simulink model "huamo"  (R2014a)
settings: Solver=ode3  SolverMode=SingleTasking  StartTime=0.0  StopTime=10.0  RelTol=1e-3
PreLoadFcn:
  | waijung.modelPreload; % Required for working with Waijung Blockset. Do not remove.
undefined symbols (not defined in the file): ARM, dfilt, DiscIntNeverNeededParam, fdesignblkfcn, gcbh, Link, LQFP64, MDK, ST, STM32F405RG
libraries: simulink x33, stm32f4_io_lib x3, stm32f4_device_config_lib x2, dsparch4 x2
(part 5 of 6)

== system huamo/ from shangweiji/Enabled Subsystem6 ==
  P : Inport
  nP : Inport  Port=2
  nI : Inport  Port=3
  nD : Inport  Port=4
  status : Inport  Port=5
  Enable : EnablePort
  UART Tx : S-Function  Priority=1  FunctionName=stm32f4_usart  Parameters=configuration,uartmodule,transfer,baudrate,inputtype,outputtype,confstr,binheaderarray,binterminatorarray,asciiheader,asciiterminator,bindatalength,packetmode,varname,sampletime,sampletimestr,blockid  EnableBusSupport=off  mask(stm32f4_usart){configuration=Tx, uartmodule=1, baudrate=115200, databits=8, parity=No, stopbit=1, remaptxpin=Not used, remaprxpin=Not used, flowcontrol=None, remapctspin=Not used, remaprtspin=Not used, advanceoptions=off, rxbuffersize=512, txbuffersize=512, transfer=Non-Blocking, packetmode=Ascii, binheader='7E 7E', binterminator='03 03', porttype_double=0, porttype_single=0, porttype_int8=0, porttype_uint8=0, porttype_int16=0, porttype_uint16=0, porttype_int32=0, porttype_uint32=3, asciiformat='alt_change_OK', rx_asciiterminator=CRLF (0x0D 0x0A - "\r\n"), tx_asciiterminator=CRLF (0x0D 0x0A - "\r\n"), storagename=<empty>, varname=, inputtype=[0 ], outputtype=[0], binheaderarray=[0], binterminatorarray=[0], bindatalength=0, asciiheader='alt_change_OK\r\n', asciiterminator=[2 13 10], sampletime=-1, sampletimestr=0.005, blockid=fromshangweijiEnabledSubsystem6UARTTx, confstr=[ "dummy", "0", "*", "*", "0", "*", "*", "0", "*", "*", "0", "*", "*", "2", "4", "7", "2", "4", "2", "512", "512", "2", "1", "115200", "8", "No", "1", "None", "USART1"], lastmodule=1}
      mask prompts: uartmodule "UART Module"; baudrate "Baud rate (bps)"; databits "Data bits"; stopbit "Stop bit"; remaptxpin "Tx Pin"; remaprxpin "Rx Pin"; flowcontrol "Hardware flow control"; remapctspin "HW Flow control, CTS Pin"; remaprtspin "HW Flow control, RTS Pin"; advanceoptions "Advance options"; rxbuffersize "Rx buffer size (bytes)"; txbuffersize "Tx buffer size (bytes)"; packetmode "Packet mode"; binheader "Binary header (example: '7E 7E')"; binterminator "Binary terminator (example: '03 03')"; porttype_double "Number of data port, type DOUBLE"; porttype_single "Number of data port, type SINGLE"; porttype_int8 "Number of data port, type INT8"; porttype_uint8 "Number of data port, type UINT8"; porttype_int16 "Number of data port, type INT16"; porttype_uint16 "Number of data port, type UINT16"; porttype_int32 "Number of data port, type INT32"; porttype_uint32 "Number of data port, type UINT32"; asciiformat "Ascii format"; rx_asciiterminator "End of packet"; tx_asciiterminator "End of packet"; storagename "Buffer"; varname "Var name"; inputtype "Input data type"; outputtype "Output data type"; binheaderarray "Binary header"; binterminatorarray "Binary terminator"; bindatalength "Binary data length"; asciiheader "Ascii header (printf format)"; asciiterminator "Ascii terminator"; sampletime "Sample time (sec)"; sampletimestr "Compiled sample time (sec) in string"; confstr "Configuration string"; lastmodule "Last module selected"
      mask help:
      | Data type for Ascii format
      | %u, %i, %d, %o, %x: uint32
      | %e, %g, %f: single
      | %c: int8
      mask init:
      | stm32f4_usart_callback('init');
      mask Help: web(fullfile(waijungdocroot,'stm32f4_usart_tx.htm'), '-browser')
      mask TypeOptions configuration: Setup | Tx | Rx
      mask Callback configuration: stm32f4_usart_callback('configuration');
      mask TypeOptions uartmodule: 1 | 2 | 3 | 4 | 5 | 6
      mask Callback uartmodule: stm32f4_usart_callback('uartmodule');
      mask Callback baudrate: stm32f4_usart_callback('baudrate');
      mask TypeOptions databits: 8
      mask TypeOptions parity: No | Odd | Even
      mask TypeOptions stopbit: 0.5 | 1 | 1.5 | 2
      mask TypeOptions remaptxpin: Not used | A9 | B6
      mask TypeOptions remaprxpin: Not used | A10 | B7
      mask TypeOptions flowcontrol: None | RTS | CTS | RTS/CTS
      mask Callback flowcontrol: stm32f4_usart_callback('flowcontrol');
      mask TypeOptions remapctspin: Not used | A11
      mask TypeOptions remaprtspin: Not used | A12
      mask Callback advanceoptions: stm32f4_usart_callback('advanceoptions');
      mask TypeOptions rxbuffersize: 16 | 32 | 64 | 128 | 256 | 512 | 1024 | 2048
      mask TypeOptions txbuffersize: 16 | 32 | 64 | 128 | 256 | 512 | 1024 | 2048
      mask TypeOptions transfer: Blocking | Non-Blocking
      mask Callback transfer: stm32f4_usart_callback('transfer');
      mask TypeOptions packetmode: Ascii | Binary | Binary Vector | String Buffer
      mask Callback packetmode: stm32f4_usart_callback('packetmode');
      mask Callback binheader: stm32f4_usart_callback('binheader');
      mask Callback binterminator: stm32f4_usart_callback('binterminator');
      mask Callback porttype_double: stm32f4_usart_callback('porttype');
      mask Callback porttype_single: stm32f4_usart_callback('porttype');
      mask Callback porttype_int8: stm32f4_usart_callback('porttype');
      mask Callback porttype_uint8: stm32f4_usart_callback('porttype');
      mask Callback porttype_int16: stm32f4_usart_callback('porttype');
      mask Callback porttype_uint16: stm32f4_usart_callback('porttype');
      mask Callback porttype_int32: stm32f4_usart_callback('porttype');
      mask Callback porttype_uint32: stm32f4_usart_callback('porttype');
      mask Callback asciiformat: stm32f4_usart_callback('asciiformat');
      mask TypeOptions rx_asciiterminator: CR (0x0D - "\r") | LF (0x0A - "\n") | CRLF (0x0D 0x0A - "\r\n")
      mask Callback rx_asciiterminator: stm32f4_usart_callback('rx_asciiterminator');
      mask TypeOptions tx_asciiterminator: CR (0x0D - "\r") | LF (0x0A - "\n") | CRLF (0x0D 0x0A - "\r\n") | None
      mask Callback tx_asciiterminator: stm32f4_usart_callback('tx_asciiterminator');
      mask TypeOptions storagename: <empty>
      mask Callback storagename: stm32f4_usart_callback('storagename');
      mask Callback varname: stm32f4_usart_callback('varname');
      mask Callback sampletime: stm32f4_usart_callback('sampletime');
      mask Callback sampletimestr: stm32f4_usart_callback('sampletimestr');
      mask Callback blockid: stm32f4_usart_callback('blockid');
      mask Display: text(0.5, 0.5, 'Module: USART1_Tx\nPacket: Ascii\nTransfer: Non-Blocking\nTs (sec): 0.005','ver','middle','hor','center');
  Out1 : Outport
  Out2 : Outport  Port=2
  Out3 : Outport  Port=3
  Out4 : Outport  Port=4
  Out5 : Outport  Port=5
  wires:
  status/1 -> Out5/1
  nD/1 -> Out4/1
  nI/1 -> Out3/1
  nP/1 -> Out2/1
  P/1 -> Out1/1

== system huamo/Controller/Angle_hold ==
  Guidance_in : Inport
  Signal_back : Inport  Port=2
  parameter_roll : Inport  Port=3
  parameter_yaw : Inport  Port=4
  parameter_alt : Inport  Port=5
  alt_back : Inport  Port=6
  Enable : EnablePort
  Bus Selector : BusSelector  OutputSignals=thrust/CH3
  Constant1 : Constant  Value=[1;1;1;1]  OutDataTypeStr=single
  Gain : Gain  Gain=[1;1;1;1]  Multiplication=Matrix(K*u)
  If : If  IfExpression=u1 > 0.2
  Subsystem : Subsystem
  Sum : Sum  Inputs=|++
  Switch : Switch  Criteria=u2 > Threshold  Threshold=0.2
  Out1 : Outport
  Out2 : Outport  Port=2
  wires:
  Bus Selector/1 -> If/1, Gain/1, Switch/2  "<thrust/CH3>"
  Gain/1 -> Switch/3
  Constant1/1 -> Sum/2
  Sum/1 -> Out1/1
  Switch/1 -> Sum/1
  alt_back/1 -> Subsystem/1(In2)
  parameter_alt/1 -> Subsystem/2(In3)
  parameter_roll/1 -> Subsystem/3(In4)
  parameter_yaw/1 -> Subsystem/4(In5)
  Guidance_in/1 -> Bus Selector/1, Subsystem/5(In6)
  Signal_back/1 -> Subsystem/6(In7)
  Subsystem/1(Out1) -> Switch/1
  Subsystem/2(Out2) -> Out2/1
  If/1 -> Subsystem/Action

== system huamo/Controller/Parameter ==
  Mux : Mux  Inputs=5
  Mux1 : Mux  Inputs=5
  Mux2 : Mux  Inputs=5
  Out1 : Outport
  Out2 : Outport  Port=2
  Out3 : Outport  Port=3
  wires:
  [roll_nD] -> Mux/4
  [yaw_nD] -> Mux1/4
  [yaw_status] -> Mux1/5
  [roll_nI] -> Mux/3
  Mux/1 -> Out1/1
  [roll_nP] -> Mux/2
  [roll_status] -> Mux/5
  [yaw_nI] -> Mux1/3
  [roll_P] -> Mux/1
  [yaw_P] -> Mux1/1
  [yaw_nP] -> Mux1/2
  Mux1/1 -> Out2/1
  [alt_nD] -> Mux2/4
  [alt_status] -> Mux2/5
  [alt_nI] -> Mux2/3
  [alt_P] -> Mux2/1
  [alt_nP] -> Mux2/2
  Mux2/1 -> Out3/1

== system huamo/Controller/Velocity_Damper1 ==
  Signal_back : Inport
  status : Inport  Port=2
  Altitude_calculation : Subsystem
  Bus Selector1 : BusSelector  OutputSignals=angle,acceleration,altitude
  Constant : Constant  Value=[0 0 9.9]
  Controller : Subsystem
  Data Type Conversion1 : DataTypeConversion  OutDataTypeStr=single
  Data Type Conversion3 : DataTypeConversion  OutDataTypeStr=double
  Digital Clock : DigitalClock  SampleTime=-1
  Digital Clock1 : DigitalClock  SampleTime=-1
  Get_initial_altitude : MATLAB Function  TreatAsAtomicUnit=on
  Horizontal_velocity : Subsystem
  If : If  IfExpression=u1 > 2  ShowElse=off
  If Action Subsystem : Subsystem  TreatAsAtomicUnit=on
  MATLAB Function : MATLAB Function  TreatAsAtomicUnit=on
  accb_to_acce : Subsystem  TreatAsAtomicUnit=on
  Alt : Outport
  Alt_rate : Outport  Port=2
  M_y : Outport  Port=3
  M_x : Outport  Port=4
  wires:
  Signal_back/1 -> Bus Selector1/1
  Altitude_calculation/1(Out1) -> Data Type Conversion3/1, Controller/1(In1)
  Bus Selector1/1 -> accb_to_acce/1(angle)  "<angle>"
  Bus Selector1/2 -> accb_to_acce/2(accel)  "<acceleration>"
  Constant/1 -> accb_to_acce/3(bias_acc)
  Get_initial_altitude/1(y) -> Altitude_calculation/3(Basic_altitude)
  Digital Clock/1 -> Get_initial_altitude/2(t)
  If Action Subsystem/1(Out1) -> Altitude_calculation/Enable
  If/1 -> If Action Subsystem/Action
  Digital Clock1/1 -> If/1
  Bus Selector1/3 -> Get_initial_altitude/1(h), Altitude_calculation/2(Barometer)  "<altitude>"
  accb_to_acce/1(Out1) -> Horizontal_velocity/1(In1), Altitude_calculation/1(Accelerometer)
  Horizontal_velocity/1(Out1) -> M_y/1
  Horizontal_velocity/2(Out2) -> M_x/1
  Data Type Conversion3/1 -> MATLAB Function/2(u2)
  MATLAB Function/1(y) -> Data Type Conversion1/1
  status/1 -> MATLAB Function/1(u1)
  Controller/1(Out1) -> Alt_rate/1
  Data Type Conversion1/1 -> Alt/1

== system huamo/Controller/Velocity_Damper2 ==
  Signal_back : Inport
  status : Inport  Port=2
  Bus Selector1 : BusSelector  OutputSignals=alt
  Controller : Subsystem
  Data Type Conversion1 : DataTypeConversion  OutDataTypeStr=single
  Data Type Conversion3 : DataTypeConversion  OutDataTypeStr=double
  Lowpass Filter : Subsystem  DialogController=fdesignblkfcn  InitFcn=fdesignblkfcn(gcbh, {'InitFcn'});  mask(Lowpass Filter){}
      mask help: Design a lowpass filter
      settings: CopyFcn=fdesignblkfcn(gcbh, {'CopyFcn'});
      mask Help: helpview(mapfilelocation('dsp'), 'dsplowpassfilter');
      mask Display: disp('Lowpass')
  MATLAB Function : MATLAB Function  TreatAsAtomicUnit=on
  Rate Transition : RateTransition
  Alt : Outport
  Alt_rate : Outport  Port=2
  wires:
  Signal_back/1 -> Bus Selector1/1
  Bus Selector1/1 -> Rate Transition/1, Data Type Conversion3/1  "<alt>"
  Data Type Conversion3/1 -> MATLAB Function/2(u2)
  MATLAB Function/1(y) -> Lowpass Filter/1(In)
  status/1 -> MATLAB Function/1(u1)
  Controller/1(Out1) -> Alt_rate/1
  Data Type Conversion1/1 -> Alt/1
  Rate Transition/1 -> Controller/1(In1)
  Lowpass Filter/1(Out) -> Data Type Conversion1/1

== system huamo/Guidance_System/Duty to Force ==
  Duty : Inport
  Add : Sum  Inputs=+-
  Constant : Constant  OutDataTypeStr=single
  Gain : Gain  OutDataTypeStr=Inherit: Same as input
  Saturation : Saturate  UpperLimit=1  LowerLimit=0
  angle : Outport
  wires:
  Add/1 -> Gain/1
  Duty/1 -> Add/1
  Constant/1 -> Add/2
  Gain/1 -> Saturation/1
  Saturation/1 -> angle/1

== system huamo/Guidance_System/Duty to angle1 ==
  Duty : Inport
  Add : Sum  Inputs=+-
  Constant : Constant  Value=1.5  OutDataTypeStr=single
  Gain : Gain  Gain=-358  OutDataTypeStr=Inherit: Same as input
  Saturation : Saturate  UpperLimit=180  LowerLimit=-180
  angle : Outport
  wires:
  Add/1 -> Gain/1
  Duty/1 -> Add/1
  Constant/1 -> Add/2
  Gain/1 -> Saturation/1
  Saturation/1 -> angle/1

== system huamo/Guidance_System/Duty to angle2 ==
  Duty : Inport
  Add : Sum  Inputs=+-
  Constant : Constant  Value=1.5  OutDataTypeStr=single
  Gain : Gain  Gain=-40  OutDataTypeStr=Inherit: Same as input
  Saturation : Saturate  UpperLimit=25  LowerLimit=-25
  angle : Outport
  wires:
  Saturation/1 -> angle/1
  Gain/1 -> Saturation/1
  Constant/1 -> Add/2
  Duty/1 -> Add/1
  Add/1 -> Gain/1

== system huamo/Guidance_System/Duty to angle3 ==
  Duty : Inport
  Add : Sum  Inputs=+-
  Constant : Constant  Value=1.5  OutDataTypeStr=single
  Gain : Gain  Gain=40  OutDataTypeStr=Inherit: Same as input
  Saturation : Saturate  UpperLimit=25  LowerLimit=-25
  angle : Outport
  wires:
  Add/1 -> Gain/1
  Duty/1 -> Add/1
  Constant/1 -> Add/2
  Gain/1 -> Saturation/1
  Saturation/1 -> angle/1

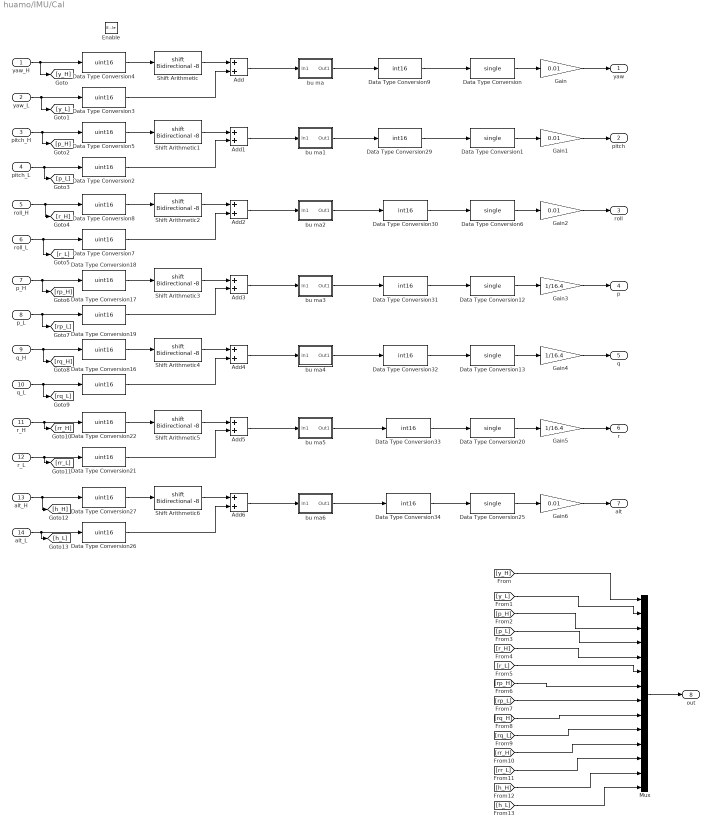
== system huamo/IMU/Cal ==
  yaw_H : Inport
  yaw_L : Inport  Port=2
  pitch_H : Inport  Port=3
  pitch_L : Inport  Port=4
  roll_H : Inport  Port=5
  roll_L : Inport  Port=6
  p_H : Inport  Port=7
  p_L : Inport  Port=8
  q_H : Inport  Port=9
  q_L : Inport  Port=10
  r_H : Inport  Port=11
  r_L : Inport  Port=12
  alt_H : Inport  Port=13
  alt_L : Inport  Port=14
  Enable : EnablePort
  Add{,1..6} (7 alike) : Sum  AccumDataTypeStr=uint16
  Data Type Conversion{,1,6,12..13,20,25} (7 alike) : DataTypeConversion  OutDataTypeStr=single
  Data Type Conversion{2..5,7..8,16..19,21..22,26..27} (14 alike) : DataTypeConversion  OutDataTypeStr=uint16
  Data Type Conversion{9,29..34} (7 alike) : DataTypeConversion  OutDataTypeStr=int16
  Gain{,1..2,6} (4 alike) : Gain  Gain=0.01
  Gain3 : Gain  Gain=1/16.4
  Gain4 : Gain  Gain=1/16.4
  Gain5 : Gain  Gain=1/16.4
  Mux : Mux  Inputs=14
  Shift Arithmetic{,1..6} (7 alike) : ArithShift  BitShiftNumber=-8
  bu ma : Subsystem
  bu ma1 : Subsystem
  bu ma2 : Subsystem
  bu ma3 : Subsystem
  bu ma4 : Subsystem
  bu ma5 : Subsystem
  bu ma6 : Subsystem
  yaw : Outport
  pitch : Outport  Port=2
  roll : Outport  Port=3
  p : Outport  Port=4
  q : Outport  Port=5
  r : Outport  Port=6
  alt : Outport  Port=7
  out : Outport  Port=8
  wires:
  Data Type Conversion/1 -> Gain/1
  yaw_H/1 -> [y_H], Data Type Conversion4/1
  yaw_L/1 -> [y_L], Data Type Conversion3/1
  Data Type Conversion1/1 -> Gain1/1
  pitch_H/1 -> [p_H], Data Type Conversion5/1
  pitch_L/1 -> [p_L], Data Type Conversion2/1
  Data Type Conversion4/1 -> Shift Arithmetic/1
  Data Type Conversion5/1 -> Shift Arithmetic1/1
  Data Type Conversion6/1 -> Gain2/1
  roll_H/1 -> [r_H], Data Type Conversion8/1
  roll_L/1 -> [r_L], Data Type Conversion7/1
  Data Type Conversion8/1 -> Shift Arithmetic2/1
  Gain/1 -> yaw/1
  Gain1/1 -> pitch/1
  Gain2/1 -> roll/1
  Data Type Conversion12/1 -> Gain3/1
  p_H/1 -> [rp_H], Data Type Conversion18/1
  p_L/1 -> [rp_L], Data Type Conversion17/1
  Data Type Conversion13/1 -> Gain4/1
  q_H/1 -> [rq_H], Data Type Conversion19/1
  q_L/1 -> [rq_L], Data Type Conversion16/1
  Data Type Conversion18/1 -> Shift Arithmetic3/1
  Data Type Conversion19/1 -> Shift Arithmetic4/1
  Data Type Conversion20/1 -> Gain5/1
  r_H/1 -> [rr_H], Data Type Conversion22/1
  r_L/1 -> [rr_L], Data Type Conversion21/1
  Data Type Conversion22/1 -> Shift Arithmetic5/1
  Gain3/1 -> p/1
  Gain4/1 -> q/1
  Gain5/1 -> r/1
  Data Type Conversion25/1 -> Gain6/1
  alt_H/1 -> [h_H], Data Type Conversion27/1
  alt_L/1 -> [h_L], Data Type Conversion26/1
  Data Type Conversion27/1 -> Shift Arithmetic6/1
  Gain6/1 -> alt/1
  Shift Arithmetic/1 -> Add/1
  Data Type Conversion3/1 -> Add/2
  Shift Arithmetic1/1 -> Add1/1
  Data Type Conversion2/1 -> Add1/2
  Shift Arithmetic2/1 -> Add2/1
  Data Type Conversion7/1 -> Add2/2
  Shift Arithmetic3/1 -> Add3/1
  Data Type Conversion17/1 -> Add3/2
  Shift Arithmetic4/1 -> Add4/1
  Data Type Conversion16/1 -> Add4/2
  Shift Arithmetic5/1 -> Add5/1
  Data Type Conversion21/1 -> Add5/2
  Shift Arithmetic6/1 -> Add6/1
  Data Type Conversion26/1 -> Add6/2
  Data Type Conversion29/1 -> Data Type Conversion1/1
  Data Type Conversion30/1 -> Data Type Conversion6/1
  Data Type Conversion31/1 -> Data Type Conversion12/1
  Data Type Conversion32/1 -> Data Type Conversion13/1
  Data Type Conversion33/1 -> Data Type Conversion20/1
  Data Type Conversion34/1 -> Data Type Conversion25/1
  Data Type Conversion9/1 -> Data Type Conversion/1
  Add/1 -> bu ma/1(In1)
  bu ma/1(Out1) -> Data Type Conversion9/1
  Add1/1 -> bu ma1/1(In1)
  bu ma1/1(Out1) -> Data Type Conversion29/1
  Add6/1 -> bu ma6/1(In1)
  bu ma6/1(Out1) -> Data Type Conversion34/1
  bu ma5/1(Out1) -> Data Type Conversion33/1
  bu ma4/1(Out1) -> Data Type Conversion32/1
  bu ma3/1(Out1) -> Data Type Conversion31/1
  bu ma2/1(Out1) -> Data Type Conversion30/1
  Add2/1 -> bu ma2/1(In1)
  Add3/1 -> bu ma3/1(In1)
  Add4/1 -> bu ma4/1(In1)
  Add5/1 -> bu ma5/1(In1)
  [y_H] -> Mux/1
  [y_L] -> Mux/2
  [p_H] -> Mux/3
  [p_L] -> Mux/4
  [r_H] -> Mux/5
  [r_L] -> Mux/6
  [rp_H] -> Mux/7
  [rp_L] -> Mux/8
  [rq_H] -> Mux/9
  [rq_L] -> Mux/10
  [rr_H] -> Mux/11
  [rr_L] -> Mux/12
  [h_H] -> Mux/13
  [h_L] -> Mux/14
  Mux/1 -> out/1

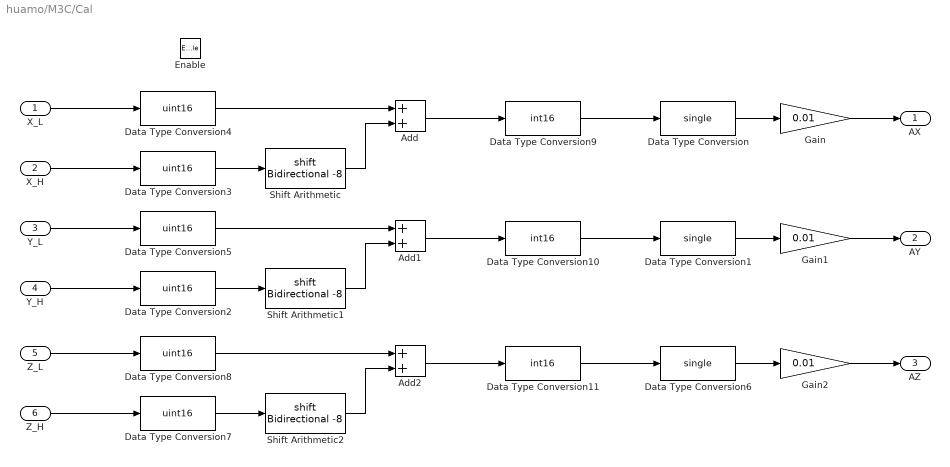
== system huamo/M3C/Cal ==
  X_L : Inport
  X_H : Inport  Port=2
  Y_L : Inport  Port=3
  Y_H : Inport  Port=4
  Z_L : Inport  Port=5
  Z_H : Inport  Port=6
  Enable : EnablePort
  Add : Sum  AccumDataTypeStr=uint16
  Add1 : Sum  AccumDataTypeStr=uint16
  Add2 : Sum  AccumDataTypeStr=uint16
  Data Type Conversion : DataTypeConversion  OutDataTypeStr=single
  Data Type Conversion1 : DataTypeConversion  OutDataTypeStr=single
  Data Type Conversion10 : DataTypeConversion  OutDataTypeStr=int16
  Data Type Conversion11 : DataTypeConversion  OutDataTypeStr=int16
  Data Type Conversion{2..5,7..8} (6 alike) : DataTypeConversion  OutDataTypeStr=uint16
  Data Type Conversion6 : DataTypeConversion  OutDataTypeStr=single
  Data Type Conversion9 : DataTypeConversion  OutDataTypeStr=int16
  Gain : Gain  Gain=0.01
  Gain1 : Gain  Gain=0.01
  Gain2 : Gain  Gain=0.01
  Shift Arithmetic : ArithShift  BitShiftNumber=-8
  Shift Arithmetic1 : ArithShift  BitShiftNumber=-8
  Shift Arithmetic2 : ArithShift  BitShiftNumber=-8
  AX : Outport
  AY : Outport  Port=2
  AZ : Outport  Port=3
  wires:
  Data Type Conversion/1 -> Gain/1
  Shift Arithmetic/1 -> Add/2
  X_L/1 -> Data Type Conversion4/1
  X_H/1 -> Data Type Conversion3/1
  Data Type Conversion3/1 -> Shift Arithmetic/1
  Add/1 -> Data Type Conversion9/1
  Data Type Conversion1/1 -> Gain1/1
  Shift Arithmetic1/1 -> Add1/2
  Y_L/1 -> Data Type Conversion5/1
  Y_H/1 -> Data Type Conversion2/1
  Data Type Conversion2/1 -> Shift Arithmetic1/1
  Add1/1 -> Data Type Conversion10/1
  Data Type Conversion4/1 -> Add/1
  Data Type Conversion5/1 -> Add1/1
  Data Type Conversion6/1 -> Gain2/1
  Shift Arithmetic2/1 -> Add2/2
  Z_L/1 -> Data Type Conversion8/1
  Z_H/1 -> Data Type Conversion7/1
  Data Type Conversion7/1 -> Shift Arithmetic2/1
  Add2/1 -> Data Type Conversion11/1
  Data Type Conversion8/1 -> Add2/1
  Gain/1 -> AX/1
  Gain1/1 -> AY/1
  Gain2/1 -> AZ/1
  Data Type Conversion9/1 -> Data Type Conversion/1
  Data Type Conversion10/1 -> Data Type Conversion1/1
  Data Type Conversion11/1 -> Data Type Conversion6/1

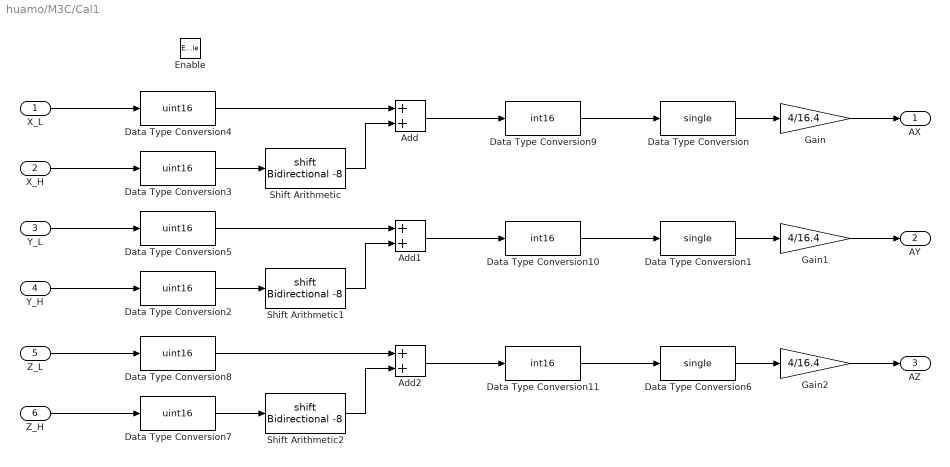
== system huamo/M3C/Cal1 ==
  X_L : Inport
  X_H : Inport  Port=2
  Y_L : Inport  Port=3
  Y_H : Inport  Port=4
  Z_L : Inport  Port=5
  Z_H : Inport  Port=6
  Enable : EnablePort
  Add : Sum  AccumDataTypeStr=uint16
  Add1 : Sum  AccumDataTypeStr=uint16
  Add2 : Sum  AccumDataTypeStr=uint16
  Data Type Conversion : DataTypeConversion  OutDataTypeStr=single
  Data Type Conversion1 : DataTypeConversion  OutDataTypeStr=single
  Data Type Conversion10 : DataTypeConversion  OutDataTypeStr=int16
  Data Type Conversion11 : DataTypeConversion  OutDataTypeStr=int16
  Data Type Conversion{2..5,7..8} (6 alike) : DataTypeConversion  OutDataTypeStr=uint16
  Data Type Conversion6 : DataTypeConversion  OutDataTypeStr=single
  Data Type Conversion9 : DataTypeConversion  OutDataTypeStr=int16
  Gain : Gain  Gain=4/16.4
  Gain1 : Gain  Gain=4/16.4
  Gain2 : Gain  Gain=4/16.4
  Shift Arithmetic : ArithShift  BitShiftNumber=-8
  Shift Arithmetic1 : ArithShift  BitShiftNumber=-8
  Shift Arithmetic2 : ArithShift  BitShiftNumber=-8
  AX : Outport
  AY : Outport  Port=2
  AZ : Outport  Port=3
  wires:
  Data Type Conversion11/1 -> Data Type Conversion6/1
  Data Type Conversion10/1 -> Data Type Conversion1/1
  Data Type Conversion9/1 -> Data Type Conversion/1
  Gain2/1 -> AZ/1
  Gain1/1 -> AY/1
  Gain/1 -> AX/1
  Data Type Conversion8/1 -> Add2/1
  Add2/1 -> Data Type Conversion11/1
  Data Type Conversion7/1 -> Shift Arithmetic2/1
  Z_H/1 -> Data Type Conversion7/1
  Z_L/1 -> Data Type Conversion8/1
  Shift Arithmetic2/1 -> Add2/2
  Data Type Conversion6/1 -> Gain2/1
  Data Type Conversion5/1 -> Add1/1
  Data Type Conversion4/1 -> Add/1
  Add1/1 -> Data Type Conversion10/1
  Data Type Conversion2/1 -> Shift Arithmetic1/1
  Y_H/1 -> Data Type Conversion2/1
  Y_L/1 -> Data Type Conversion5/1
  Shift Arithmetic1/1 -> Add1/2
  Data Type Conversion1/1 -> Gain1/1
  Add/1 -> Data Type Conversion9/1
  Data Type Conversion3/1 -> Shift Arithmetic/1
  X_H/1 -> Data Type Conversion3/1
  X_L/1 -> Data Type Conversion4/1
  Shift Arithmetic/1 -> Add/2
  Data Type Conversion/1 -> Gain/1

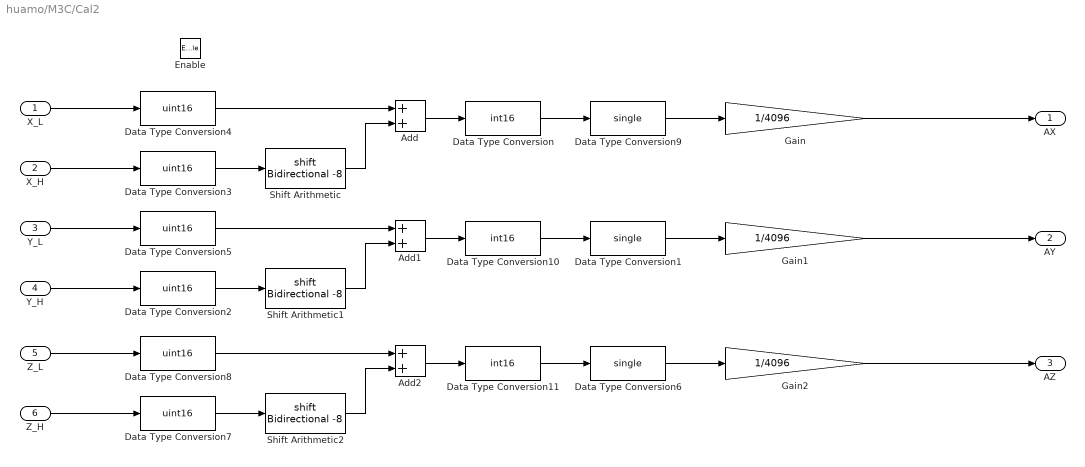
== system huamo/M3C/Cal2 ==
  X_L : Inport
  X_H : Inport  Port=2
  Y_L : Inport  Port=3
  Y_H : Inport  Port=4
  Z_L : Inport  Port=5
  Z_H : Inport  Port=6
  Enable : EnablePort
  Add : Sum
  Add1 : Sum
  Add2 : Sum
  Data Type Conversion : DataTypeConversion  OutDataTypeStr=int16
  Data Type Conversion1 : DataTypeConversion  OutDataTypeStr=single
  Data Type Conversion10 : DataTypeConversion  OutDataTypeStr=int16
  Data Type Conversion11 : DataTypeConversion  OutDataTypeStr=int16
  Data Type Conversion{2..5,7..8} (6 alike) : DataTypeConversion  OutDataTypeStr=uint16
  Data Type Conversion6 : DataTypeConversion  OutDataTypeStr=single
  Data Type Conversion9 : DataTypeConversion  OutDataTypeStr=single
  Gain : Gain  Gain=1/4096
  Gain1 : Gain  Gain=1/4096
  Gain2 : Gain  Gain=1/4096
  Shift Arithmetic : ArithShift  BitShiftNumber=-8
  Shift Arithmetic1 : ArithShift  BitShiftNumber=-8
  Shift Arithmetic2 : ArithShift  BitShiftNumber=-8
  AX : Outport
  AY : Outport  Port=2
  AZ : Outport  Port=3
  wires:
  Shift Arithmetic/1 -> Add/2
  X_L/1 -> Data Type Conversion4/1
  X_H/1 -> Data Type Conversion3/1
  Data Type Conversion3/1 -> Shift Arithmetic/1
  Add/1 -> Data Type Conversion/1
  Shift Arithmetic1/1 -> Add1/2
  Y_L/1 -> Data Type Conversion5/1
  Y_H/1 -> Data Type Conversion2/1
  Data Type Conversion2/1 -> Shift Arithmetic1/1
  Add1/1 -> Data Type Conversion10/1
  Data Type Conversion4/1 -> Add/1
  Data Type Conversion5/1 -> Add1/1
  Shift Arithmetic2/1 -> Add2/2
  Z_L/1 -> Data Type Conversion8/1
  Z_H/1 -> Data Type Conversion7/1
  Data Type Conversion7/1 -> Shift Arithmetic2/1
  Add2/1 -> Data Type Conversion11/1
  Data Type Conversion8/1 -> Add2/1
  Data Type Conversion/1 -> Data Type Conversion9/1
  Data Type Conversion1/1 -> Gain1/1
  Data Type Conversion6/1 -> Gain2/1
  Data Type Conversion9/1 -> Gain/1
  Data Type Conversion10/1 -> Data Type Conversion1/1
  Data Type Conversion11/1 -> Data Type Conversion6/1
  Gain/1 -> AX/1
  Gain1/1 -> AY/1
  Gain2/1 -> AZ/1

== system huamo/M3C/Cal3 ==
  L : Inport
  LH : Inport  Port=2
  HL : Inport  Port=3
  H : Inport  Port=4
  Enable : EnablePort
  Add : Sum  Inputs=++++
  Data Type Conversion : DataTypeConversion  OutDataTypeStr=int32
  Data Type Conversion{2..5} (4 alike) : DataTypeConversion  OutDataTypeStr=uint16
  Data Type Conversion9 : DataTypeConversion  OutDataTypeStr=single
  Gain : Gain  Gain=0.01
  Shift Arithmetic : ArithShift  BitShiftNumber=-8
  Shift Arithmetic1 : ArithShift  BitShiftNumber=-8
  Shift Arithmetic2 : ArithShift  BitShiftNumber=-8
  Altitude : Outport
  wires:
  Gain/1 -> Altitude/1
  Data Type Conversion9/1 -> Gain/1
  Data Type Conversion/1 -> Data Type Conversion9/1
  Data Type Conversion4/1 -> Add/1
  Data Type Conversion2/1 -> Shift Arithmetic1/1
  H/1 -> Data Type Conversion2/1
  HL/1 -> Data Type Conversion5/1
  Add/1 -> Data Type Conversion/1
  Data Type Conversion3/1 -> Shift Arithmetic/1
  LH/1 -> Data Type Conversion3/1
  L/1 -> Data Type Conversion4/1
  Shift Arithmetic/1 -> Add/2
  Data Type Conversion5/1 -> Shift Arithmetic2/1
  Shift Arithmetic2/1 -> Add/3
  Shift Arithmetic1/1 -> Add/4

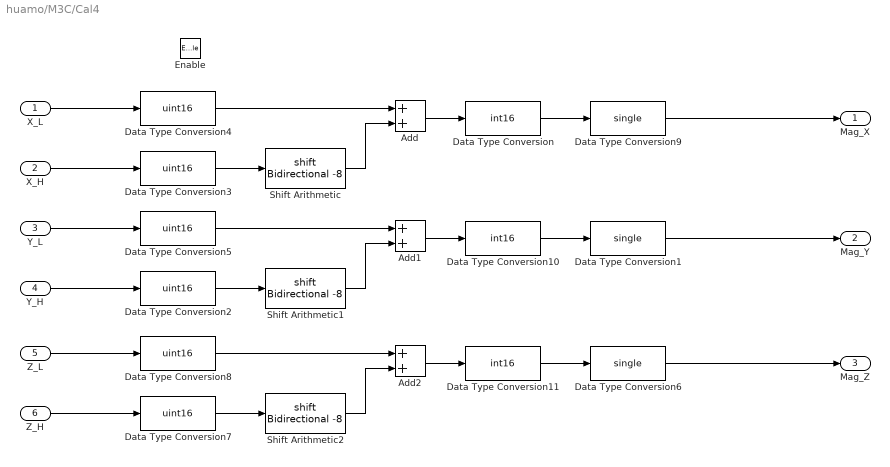
== system huamo/M3C/Cal4 ==
  X_L : Inport
  X_H : Inport  Port=2
  Y_L : Inport  Port=3
  Y_H : Inport  Port=4
  Z_L : Inport  Port=5
  Z_H : Inport  Port=6
  Enable : EnablePort
  Add : Sum
  Add1 : Sum
  Add2 : Sum
  Data Type Conversion : DataTypeConversion  OutDataTypeStr=int16
  Data Type Conversion1 : DataTypeConversion  OutDataTypeStr=single
  Data Type Conversion10 : DataTypeConversion  OutDataTypeStr=int16
  Data Type Conversion11 : DataTypeConversion  OutDataTypeStr=int16
  Data Type Conversion{2..5,7..8} (6 alike) : DataTypeConversion  OutDataTypeStr=uint16
  Data Type Conversion6 : DataTypeConversion  OutDataTypeStr=single
  Data Type Conversion9 : DataTypeConversion  OutDataTypeStr=single
  Shift Arithmetic : ArithShift  BitShiftNumber=-8
  Shift Arithmetic1 : ArithShift  BitShiftNumber=-8
  Shift Arithmetic2 : ArithShift  BitShiftNumber=-8
  Mag_X : Outport
  Mag_Y : Outport  Port=2
  Mag_Z : Outport  Port=3
  wires:
  Shift Arithmetic/1 -> Add/2
  X_L/1 -> Data Type Conversion4/1
  X_H/1 -> Data Type Conversion3/1
  Data Type Conversion3/1 -> Shift Arithmetic/1
  Add/1 -> Data Type Conversion/1
  Shift Arithmetic1/1 -> Add1/2
  Y_L/1 -> Data Type Conversion5/1
  Y_H/1 -> Data Type Conversion2/1
  Data Type Conversion2/1 -> Shift Arithmetic1/1
  Add1/1 -> Data Type Conversion10/1
  Data Type Conversion4/1 -> Add/1
  Data Type Conversion5/1 -> Add1/1
  Shift Arithmetic2/1 -> Add2/2
  Z_L/1 -> Data Type Conversion8/1
  Z_H/1 -> Data Type Conversion7/1
  Data Type Conversion7/1 -> Shift Arithmetic2/1
  Add2/1 -> Data Type Conversion11/1
  Data Type Conversion8/1 -> Add2/1
  Data Type Conversion/1 -> Data Type Conversion9/1
  Data Type Conversion1/1 -> Mag_Y/1
  Data Type Conversion6/1 -> Mag_Z/1
  Data Type Conversion10/1 -> Data Type Conversion1/1
  Data Type Conversion11/1 -> Data Type Conversion6/1
  Data Type Conversion9/1 -> Mag_X/1

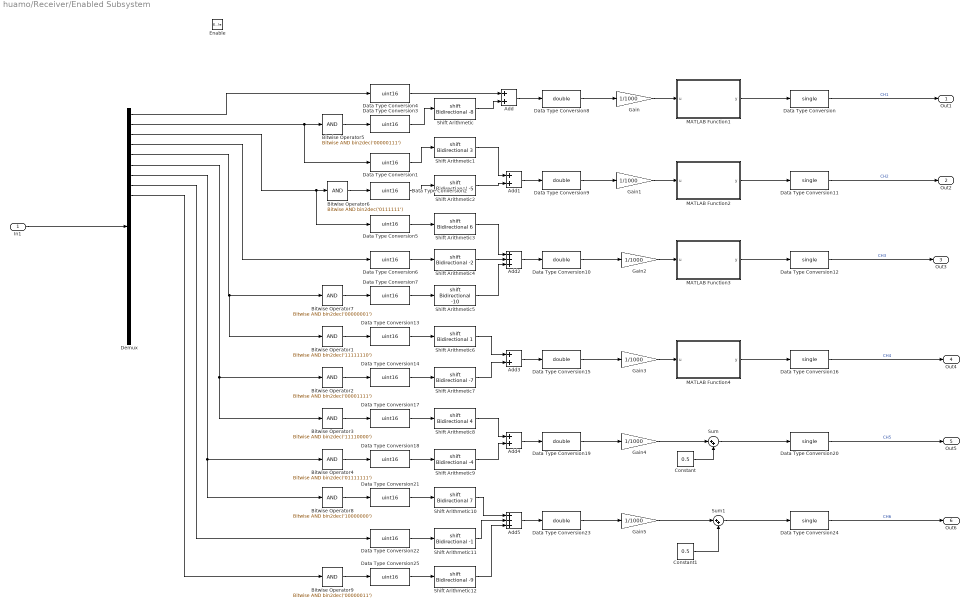
== system huamo/Receiver/Enabled Subsystem ==
  In1 : Inport
  Enable : EnablePort
  Add{,1,3..4} (4 alike) : Sum  AccumDataTypeStr=uint16
  Add2 : Sum  Inputs=+++  AccumDataTypeStr=uint16
  Add5 : Sum  Inputs=+++  AccumDataTypeStr=uint16
  Bitwise Operator1 : simulink/Logic and Bit Operations/Bitwise Operator  logicop=AND  UseBitMask=on  BitMask=bin2dec('11111110')  BitMaskRealWorld=Stored Integer
  Bitwise Operator2 : simulink/Logic and Bit Operations/Bitwise Operator  logicop=AND  UseBitMask=on  BitMask=bin2dec('00001111')  BitMaskRealWorld=Stored Integer
  Bitwise Operator3 : simulink/Logic and Bit Operations/Bitwise Operator  logicop=AND  UseBitMask=on  BitMask=bin2dec('11110000')  BitMaskRealWorld=Stored Integer
  Bitwise Operator4 : simulink/Logic and Bit Operations/Bitwise Operator  logicop=AND  UseBitMask=on  BitMask=bin2dec('01111111')  BitMaskRealWorld=Stored Integer
  Bitwise Operator5 : simulink/Logic and Bit Operations/Bitwise Operator  logicop=AND  UseBitMask=on  BitMask=bin2dec('00000111')  BitMaskRealWorld=Stored Integer
  Bitwise Operator6 : simulink/Logic and Bit Operations/Bitwise Operator  logicop=AND  UseBitMask=on  BitMask=bin2dec('0111111')  BitMaskRealWorld=Stored Integer
  Bitwise Operator7 : simulink/Logic and Bit Operations/Bitwise Operator  logicop=AND  UseBitMask=on  BitMask=bin2dec('00000001')  BitMaskRealWorld=Stored Integer
  Bitwise Operator8 : simulink/Logic and Bit Operations/Bitwise Operator  logicop=AND  UseBitMask=on  BitMask=bin2dec('10000000')  BitMaskRealWorld=Stored Integer
  Bitwise Operator9 : simulink/Logic and Bit Operations/Bitwise Operator  logicop=AND  UseBitMask=on  BitMask=bin2dec('00000011')  BitMaskRealWorld=Stored Integer
  Constant : Constant  Value=0.5
  Constant1 : Constant  Value=0.5
  Data Type Conversion{,11..12,16,20,24} (6 alike) : DataTypeConversion  OutDataTypeStr=single
  Data Type Conversion{1..7,13..14,17..18,21..22,25} (14 alike) : DataTypeConversion  OutDataTypeStr=uint16
  Data Type Conversion{8..10,15,19,23} (6 alike) : DataTypeConversion  OutDataTypeStr=double
  Demux : Demux  Outputs=23
  Gain{,1..5} (6 alike) : Gain  Gain=1/1000
  MATLAB Function1 : MATLAB Function  TreatAsAtomicUnit=on
  MATLAB Function2 : MATLAB Function  TreatAsAtomicUnit=on
  MATLAB Function3 : MATLAB Function  TreatAsAtomicUnit=on
  MATLAB Function4 : MATLAB Function  TreatAsAtomicUnit=on
  Shift Arithmetic : ArithShift  BitShiftNumber=-8
  Shift Arithmetic1 : ArithShift  BitShiftNumber=3
  Shift Arithmetic10 : ArithShift  BitShiftNumber=7
  Shift Arithmetic11 : ArithShift  BitShiftNumber=-1
  Shift Arithmetic12 : ArithShift  BitShiftNumber=-9
  Shift Arithmetic2 : ArithShift  BitShiftNumber=-5
  Shift Arithmetic3 : ArithShift  BitShiftNumber=6
  Shift Arithmetic4 : ArithShift  BitShiftNumber=-2
  Shift Arithmetic5 : ArithShift  BitShiftNumber=-10
  Shift Arithmetic6 : ArithShift  BitShiftNumber=1
  Shift Arithmetic7 : ArithShift  BitShiftNumber=-7
  Shift Arithmetic8 : ArithShift  BitShiftNumber=4
  Shift Arithmetic9 : ArithShift  BitShiftNumber=-4
  Sum : Sum  Inputs=|++
  Sum1 : Sum  Inputs=|++
  Out1 : Outport
  Out2 : Outport  Port=2
  Out3 : Outport  Port=3
  Out4 : Outport  Port=4
  Out5 : Outport  Port=5
  Out6 : Outport  Port=6
  wires:
  Data Type Conversion4/1 -> Add/1
  Data Type Conversion3/1 -> Shift Arithmetic/1
  Shift Arithmetic/1 -> Add/2
  Demux/1 -> Data Type Conversion4/1
  Bitwise Operator5/1 -> Data Type Conversion3/1
  Data Type Conversion1/1 -> Shift Arithmetic1/1
  Demux/2 -> Data Type Conversion1/1, Bitwise Operator5/1
  Data Type Conversion2/1 -> Shift Arithmetic2/1
  Shift Arithmetic1/1 -> Add1/1
  Shift Arithmetic2/1 -> Add1/2
  Data Type Conversion5/1 -> Shift Arithmetic3/1
  Demux/4 -> Data Type Conversion6/1
  Data Type Conversion6/1 -> Shift Arithmetic4/1
  Data Type Conversion7/1 -> Shift Arithmetic5/1
  Shift Arithmetic3/1 -> Add2/1
  Shift Arithmetic4/1 -> Add2/2
  Shift Arithmetic5/1 -> Add2/3
  Add1/1 -> Data Type Conversion9/1
  Add2/1 -> Data Type Conversion10/1
  Data Type Conversion10/1 -> Gain2/1
  Gain/1 -> MATLAB Function1/1(u)
  Gain1/1 -> MATLAB Function2/1(u)
  Gain2/1 -> MATLAB Function3/1(u)
  Data Type Conversion/1 -> Out1/1  "CH1"
  Data Type Conversion11/1 -> Out2/1  "CH2"
  Data Type Conversion12/1 -> Out3/1  "CH3"
  In1/1 -> Demux/1
  Demux/3 -> Bitwise Operator6/1, Data Type Conversion5/1
  Bitwise Operator6/1 -> Data Type Conversion2/1
  Bitwise Operator7/1 -> Data Type Conversion7/1
  Demux/5 -> Bitwise Operator1/1, Bitwise Operator7/1
  Bitwise Operator1/1 -> Data Type Conversion13/1
  Data Type Conversion13/1 -> Shift Arithmetic6/1
  Demux/6 -> Bitwise Operator3/1, Bitwise Operator2/1
  Bitwise Operator2/1 -> Data Type Conversion14/1
  Data Type Conversion14/1 -> Shift Arithmetic7/1
  Shift Arithmetic6/1 -> Add3/1
  Shift Arithmetic7/1 -> Add3/2
  Add3/1 -> Data Type Conversion15/1
  Data Type Conversion15/1 -> Gain3/1
  Gain3/1 -> MATLAB Function4/1(u)
  Bitwise Operator3/1 -> Data Type Conversion17/1
  Data Type Conversion17/1 -> Shift Arithmetic8/1
  Bitwise Operator4/1 -> Data Type Conversion18/1
  Data Type Conversion18/1 -> Shift Arithmetic9/1
  Shift Arithmetic8/1 -> Add4/1
  Shift Arithmetic9/1 -> Add4/2
  Add4/1 -> Data Type Conversion19/1
  Demux/7 -> Bitwise Operator8/1, Bitwise Operator4/1
  Data Type Conversion19/1 -> Gain4/1
  Bitwise Operator8/1 -> Data Type Conversion21/1
  Data Type Conversion21/1 -> Shift Arithmetic10/1
  Demux/8 -> Data Type Conversion22/1
  Data Type Conversion22/1 -> Shift Arithmetic11/1
  Shift Arithmetic10/1 -> Add5/1
  Shift Arithmetic11/1 -> Add5/2
  Add5/1 -> Data Type Conversion23/1
  Data Type Conversion23/1 -> Gain5/1
  Data Type Conversion25/1 -> Shift Arithmetic12/1
  Shift Arithmetic12/1 -> Add5/3
  Bitwise Operator9/1 -> Data Type Conversion25/1
  Demux/9 -> Bitwise Operator9/1
  Data Type Conversion16/1 -> Out4/1  "CH4"
  Data Type Conversion20/1 -> Out5/1  "CH5"
  Data Type Conversion24/1 -> Out6/1  "CH6"
  Add/1 -> Data Type Conversion8/1
  Data Type Conversion8/1 -> Gain/1
  Data Type Conversion9/1 -> Gain1/1
  MATLAB Function1/1(y) -> Data Type Conversion/1
  MATLAB Function4/1(y) -> Data Type Conversion16/1
  MATLAB Function2/1(y) -> Data Type Conversion11/1
  Gain4/1 -> Sum/1
  Sum/1 -> Data Type Conversion20/1
  Constant/1 -> Sum/2
  Sum1/1 -> Data Type Conversion24/1
  Gain5/1 -> Sum1/1
  Constant1/1 -> Sum1/2
  MATLAB Function3/1(y) -> Data Type Conversion12/1

== system huamo/to shangweiji/Subsystem ==
  In3 : Inport
  Demux : Demux  Outputs=5
  UART Tx : S-Function  Priority=1  FunctionName=stm32f4_usart  Parameters=configuration,uartmodule,transfer,baudrate,inputtype,outputtype,confstr,binheaderarray,binterminatorarray,asciiheader,asciiterminator,bindatalength,packetmode,varname,sampletime,sampletimestr,blockid  EnableBusSupport=off  mask(stm32f4_usart){configuration=Tx, uartmodule=1, baudrate=115200, databits=8, parity=No, stopbit=1, remaptxpin=Not used, remaprxpin=Not used, flowcontrol=None, remapctspin=Not used, remaprtspin=Not used, advanceoptions=off, rxbuffersize=512, txbuffersize=512, transfer=Non-Blocking, packetmode=Ascii, binheader='7E 7E', binterminator='03 03', porttype_double=0, porttype_single=0, porttype_int8=0, porttype_uint8=23, porttype_int16=0, porttype_uint16=0, porttype_int32=0, porttype_uint32=0, asciiformat='dianji=%f,%f,%f,%f,%f', rx_asciiterminator=CRLF (0x0D 0x0A - "\r\n"), tx_asciiterminator=CRLF (0x0D 0x0A - "\r\n"), storagename=<empty>, varname=, inputtype=[5  1 1 1 1 1], outputtype=[0], binheaderarray=[0], binterminatorarray=[0], bindatalength=0, asciiheader='dianji=%f,%f,%f,%f,%f\r\n', asciiterminator=[2 13 10], sampletime=-1, sampletimestr=0.6, blockid=toshangweijiSubsystemUARTTx, confstr=[ "dummy", "0", "*", "*", "0", "*", "*", "0", "*", "*", "0", "*", "*", "2", "4", "7", "2", "4", "2", "512", "512", "2", "1", "115200", "8", "No", "1", "None", "USART1"], lastmodule=1}
      mask prompts: uartmodule "UART Module"; baudrate "Baud rate (bps)"; databits "Data bits"; stopbit "Stop bit"; remaptxpin "Tx Pin"; remaprxpin "Rx Pin"; flowcontrol "Hardware flow control"; remapctspin "HW Flow control, CTS Pin"; remaprtspin "HW Flow control, RTS Pin"; advanceoptions "Advance options"; rxbuffersize "Rx buffer size (bytes)"; txbuffersize "Tx buffer size (bytes)"; packetmode "Packet mode"; binheader "Binary header (example: '7E 7E')"; binterminator "Binary terminator (example: '03 03')"; porttype_double "Number of data port, type DOUBLE"; porttype_single "Number of data port, type SINGLE"; porttype_int8 "Number of data port, type INT8"; porttype_uint8 "Number of data port, type UINT8"; porttype_int16 "Number of data port, type INT16"; porttype_uint16 "Number of data port, type UINT16"; porttype_int32 "Number of data port, type INT32"; porttype_uint32 "Number of data port, type UINT32"; asciiformat "Ascii format"; rx_asciiterminator "End of packet"; tx_asciiterminator "End of packet"; storagename "Buffer"; varname "Var name"; inputtype "Input data type"; outputtype "Output data type"; binheaderarray "Binary header"; binterminatorarray "Binary terminator"; bindatalength "Binary data length"; asciiheader "Ascii header (printf format)"; asciiterminator "Ascii terminator"; sampletime "Sample time (sec)"; sampletimestr "Compiled sample time (sec) in string"; confstr "Configuration string"; lastmodule "Last module selected"
      mask help:
      | Data type for Ascii format
      | %u, %i, %d, %o, %x: uint32
      | %e, %g, %f: single
      | %c: int8
      mask init:
      | stm32f4_usart_callback('init');
      mask Help: web(fullfile(waijungdocroot,'stm32f4_usart_tx.htm'), '-browser')
      mask TypeOptions configuration: Setup | Tx | Rx
      mask Callback configuration: stm32f4_usart_callback('configuration');
      mask TypeOptions uartmodule: 1 | 2 | 3 | 4 | 5 | 6
      mask Callback uartmodule: stm32f4_usart_callback('uartmodule');
      mask Callback baudrate: stm32f4_usart_callback('baudrate');
      mask TypeOptions databits: 8
      mask TypeOptions parity: No | Odd | Even
      mask TypeOptions stopbit: 0.5 | 1 | 1.5 | 2
      mask TypeOptions remaptxpin: Not used | A9 | B6
      mask TypeOptions remaprxpin: Not used | A10 | B7
      mask TypeOptions flowcontrol: None | RTS | CTS | RTS/CTS
      mask Callback flowcontrol: stm32f4_usart_callback('flowcontrol');
      mask TypeOptions remapctspin: Not used | A11
      mask TypeOptions remaprtspin: Not used | A12
      mask Callback advanceoptions: stm32f4_usart_callback('advanceoptions');
      mask TypeOptions rxbuffersize: 16 | 32 | 64 | 128 | 256 | 512 | 1024 | 2048
      mask TypeOptions txbuffersize: 16 | 32 | 64 | 128 | 256 | 512 | 1024 | 2048
      mask TypeOptions transfer: Blocking | Non-Blocking
      mask Callback transfer: stm32f4_usart_callback('transfer');
      mask TypeOptions packetmode: Ascii | Binary | Binary Vector | String Buffer
      mask Callback packetmode: stm32f4_usart_callback('packetmode');
      mask Callback binheader: stm32f4_usart_callback('binheader');
      mask Callback binterminator: stm32f4_usart_callback('binterminator');
      mask Callback porttype_double: stm32f4_usart_callback('porttype');
      mask Callback porttype_single: stm32f4_usart_callback('porttype');
      mask Callback porttype_int8: stm32f4_usart_callback('porttype');
      mask Callback porttype_uint8: stm32f4_usart_callback('porttype');
      mask Callback porttype_int16: stm32f4_usart_callback('porttype');
      mask Callback porttype_uint16: stm32f4_usart_callback('porttype');
      mask Callback porttype_int32: stm32f4_usart_callback('porttype');
      mask Callback porttype_uint32: stm32f4_usart_callback('porttype');
      mask Callback asciiformat: stm32f4_usart_callback('asciiformat');
      mask TypeOptions rx_asciiterminator: CR (0x0D - "\r") | LF (0x0A - "\n") | CRLF (0x0D 0x0A - "\r\n")
      mask Callback rx_asciiterminator: stm32f4_usart_callback('rx_asciiterminator');
      mask TypeOptions tx_asciiterminator: CR (0x0D - "\r") | LF (0x0A - "\n") | CRLF (0x0D 0x0A - "\r\n") | None
      mask Callback tx_asciiterminator: stm32f4_usart_callback('tx_asciiterminator');
      mask TypeOptions storagename: <empty>
      mask Callback storagename: stm32f4_usart_callback('storagename');
      mask Callback varname: stm32f4_usart_callback('varname');
      mask Callback sampletime: stm32f4_usart_callback('sampletime');
      mask Callback sampletimestr: stm32f4_usart_callback('sampletimestr');
      mask Callback blockid: stm32f4_usart_callback('blockid');
      mask Display: text(0.5, 0.5, 'Module: USART1_Tx\nPacket: Ascii\nTransfer: Non-Blocking\nTs (sec): 0.6','ver','middle','hor','center'); port_label('input', 1,'single'); port_label('input', 2,'single'); port_label('input', 3,'single'); port_label('input', 4,'single'); port_label('input', 5,'single');
  wires:
  Demux/1 -> UART Tx/1
  Demux/2 -> UART Tx/2
  Demux/3 -> UART Tx/3
  Demux/4 -> UART Tx/4
  In3/1 -> Demux/1
  Demux/5 -> UART Tx/5

== system huamo/ from shangweiji/Enabled Subsystem1/If Action Subsystem ==
  Action Port : ActionPort  ActionType=then
  UART Tx : S-Function  Priority=1  FunctionName=stm32f4_usart  Parameters=configuration,uartmodule,transfer,baudrate,inputtype,outputtype,confstr,binheaderarray,binterminatorarray,asciiheader,asciiterminator,bindatalength,packetmode,varname,sampletime,sampletimestr,blockid  EnableBusSupport=off  mask(stm32f4_usart){configuration=Tx, uartmodule=1, baudrate=115200, databits=8, parity=No, stopbit=1, remaptxpin=Not used, remaprxpin=Not used, flowcontrol=None, remapctspin=Not used, remaprtspin=Not used, advanceoptions=off, rxbuffersize=512, txbuffersize=512, transfer=Non-Blocking, packetmode=Ascii, binheader='7E 7E', binterminator='03 03', porttype_double=0, porttype_single=0, porttype_int8=0, porttype_uint8=0, porttype_int16=0, porttype_uint16=0, porttype_int32=0, porttype_uint32=3, asciiformat='>>LED1 OFF', rx_asciiterminator=CRLF (0x0D 0x0A - "\r\n"), tx_asciiterminator=CRLF (0x0D 0x0A - "\r\n"), storagename=<empty>, varname=, inputtype=[0 ], outputtype=[0], binheaderarray=[0], binterminatorarray=[0], bindatalength=0, asciiheader='>>LED1 OFF\r\n', asciiterminator=[2 13 10], sampletime=1, sampletimestr=1, blockid=fromshangweijiEnabledSubsystem1IfActionSubsystemUARTTx, confstr=[ "dummy", "0", "*", "*", "0", "*", "*", "0", "*", "*", "0", "*", "*", "2", "4", "7", "2", "4", "2", "512", "512", "2", "1", "115200", "8", "No", "1", "None", "USART1"], lastmodule=1}
      mask prompts: uartmodule "UART Module"; baudrate "Baud rate (bps)"; databits "Data bits"; stopbit "Stop bit"; remaptxpin "Tx Pin"; remaprxpin "Rx Pin"; flowcontrol "Hardware flow control"; remapctspin "HW Flow control, CTS Pin"; remaprtspin "HW Flow control, RTS Pin"; advanceoptions "Advance options"; rxbuffersize "Rx buffer size (bytes)"; txbuffersize "Tx buffer size (bytes)"; packetmode "Packet mode"; binheader "Binary header (example: '7E 7E')"; binterminator "Binary terminator (example: '03 03')"; porttype_double "Number of data port, type DOUBLE"; porttype_single "Number of data port, type SINGLE"; porttype_int8 "Number of data port, type INT8"; porttype_uint8 "Number of data port, type UINT8"; porttype_int16 "Number of data port, type INT16"; porttype_uint16 "Number of data port, type UINT16"; porttype_int32 "Number of data port, type INT32"; porttype_uint32 "Number of data port, type UINT32"; asciiformat "Ascii format"; rx_asciiterminator "End of packet"; tx_asciiterminator "End of packet"; storagename "Buffer"; varname "Var name"; inputtype "Input data type"; outputtype "Output data type"; binheaderarray "Binary header"; binterminatorarray "Binary terminator"; bindatalength "Binary data length"; asciiheader "Ascii header (printf format)"; asciiterminator "Ascii terminator"; sampletime "Sample time (sec)"; sampletimestr "Compiled sample time (sec) in string"; confstr "Configuration string"; lastmodule "Last module selected"
      mask help:
      | Data type for Ascii format
      | %u, %i, %d, %o, %x: uint32
      | %e, %g, %f: single
      | %c: int8
      mask init:
      | stm32f4_usart_callback('init');
      mask Help: web(fullfile(waijungdocroot,'stm32f4_usart_tx.htm'), '-browser')
      mask TypeOptions configuration: Setup | Tx | Rx
      mask Callback configuration: stm32f4_usart_callback('configuration');
      mask TypeOptions uartmodule: 1 | 2 | 3 | 4 | 5 | 6
      mask Callback uartmodule: stm32f4_usart_callback('uartmodule');
      mask Callback baudrate: stm32f4_usart_callback('baudrate');
      mask TypeOptions databits: 8
      mask TypeOptions parity: No | Odd | Even
      mask TypeOptions stopbit: 0.5 | 1 | 1.5 | 2
      mask TypeOptions remaptxpin: Not used | A9 | B6
      mask TypeOptions remaprxpin: Not used | A10 | B7
      mask TypeOptions flowcontrol: None | RTS | CTS | RTS/CTS
      mask Callback flowcontrol: stm32f4_usart_callback('flowcontrol');
      mask TypeOptions remapctspin: Not used | A11
      mask TypeOptions remaprtspin: Not used | A12
      mask Callback advanceoptions: stm32f4_usart_callback('advanceoptions');
      mask TypeOptions rxbuffersize: 16 | 32 | 64 | 128 | 256 | 512 | 1024 | 2048
      mask TypeOptions txbuffersize: 16 | 32 | 64 | 128 | 256 | 512 | 1024 | 2048
      mask TypeOptions transfer: Blocking | Non-Blocking
      mask Callback transfer: stm32f4_usart_callback('transfer');
      mask TypeOptions packetmode: Ascii | Binary | Binary Vector | String Buffer
      mask Callback packetmode: stm32f4_usart_callback('packetmode');
      mask Callback binheader: stm32f4_usart_callback('binheader');
      mask Callback binterminator: stm32f4_usart_callback('binterminator');
      mask Callback porttype_double: stm32f4_usart_callback('porttype');
      mask Callback porttype_single: stm32f4_usart_callback('porttype');
      mask Callback porttype_int8: stm32f4_usart_callback('porttype');
      mask Callback porttype_uint8: stm32f4_usart_callback('porttype');
      mask Callback porttype_int16: stm32f4_usart_callback('porttype');
      mask Callback porttype_uint16: stm32f4_usart_callback('porttype');
      mask Callback porttype_int32: stm32f4_usart_callback('porttype');
      mask Callback porttype_uint32: stm32f4_usart_callback('porttype');
      mask Callback asciiformat: stm32f4_usart_callback('asciiformat');
      mask TypeOptions rx_asciiterminator: CR (0x0D - "\r") | LF (0x0A - "\n") | CRLF (0x0D 0x0A - "\r\n")
      mask Callback rx_asciiterminator: stm32f4_usart_callback('rx_asciiterminator');
      mask TypeOptions tx_asciiterminator: CR (0x0D - "\r") | LF (0x0A - "\n") | CRLF (0x0D 0x0A - "\r\n") | None
      mask Callback tx_asciiterminator: stm32f4_usart_callback('tx_asciiterminator');
      mask TypeOptions storagename: <empty>
      mask Callback storagename: stm32f4_usart_callback('storagename');
      mask Callback varname: stm32f4_usart_callback('varname');
      mask Callback sampletime: stm32f4_usart_callback('sampletime');
      mask Callback sampletimestr: stm32f4_usart_callback('sampletimestr');
      mask Callback blockid: stm32f4_usart_callback('blockid');
      mask Display: text(0.5, 0.5, 'Module: USART1_Tx\nPacket: Ascii\nTransfer: Non-Blocking\nTs (sec): 1','ver','middle','hor','center');
